simulink model "diff_drive_motion_model"  (R2018b)
settings: Solver=FixedStepDiscrete  StartTime=0.0  StopTime=10.0  FixedStep=0.01  RelTol=1e-3
values from neighbouring files (symbols this model uses):
  J = 0.02    [diff_drive_mm_workspace.m]
  K = 5    [diff_drive_mm_workspace.m]
  Kb = 0.1    [diff_drive_mm_workspace.m]
  Kf = 0.2    [diff_drive_mm_workspace.m]
  Km = 0.1    [diff_drive_mm_workspace.m]
  L = 0.5    [diff_drive_mm_workspace.m]
  R = 2.0    (= 2)    [diff_drive_mm_workspace.m]
undefined symbols (not defined in the file or in its folder): DiscIntNeverNeededParam
libraries: simulink x3
settings Model: Creator=Adhiti  LastModifiedBy=Adhiti

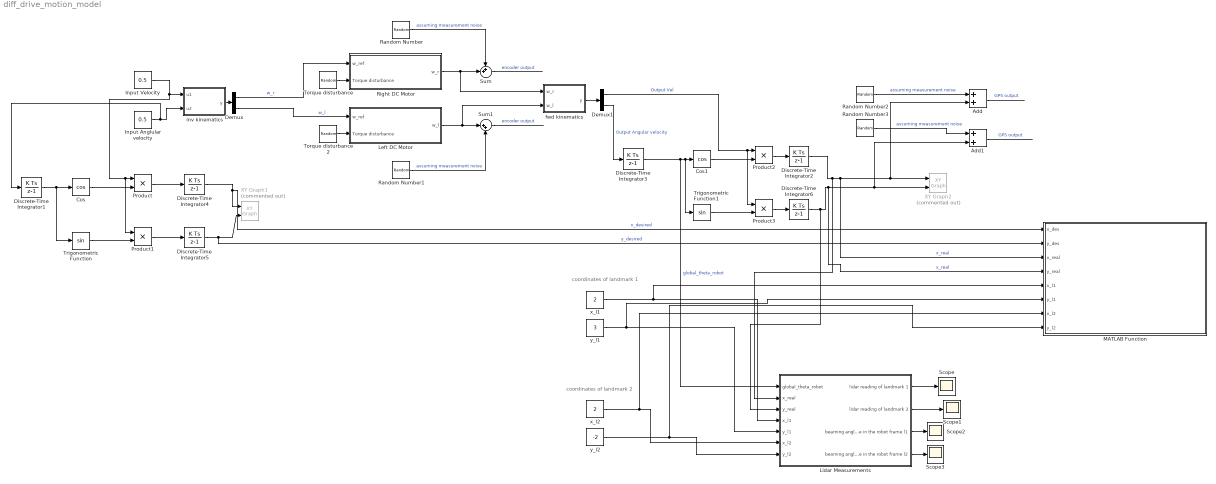
== system diff_drive_motion_model ==
  note: coordinates of landmark 2
  note: coordinates of landmark 1
  Add : Sum
  Add1 : Sum
  Cos : Trigonometry  Operator=cos
  Cos1 : Trigonometry  Operator=cos
  Demux : Demux  Outputs=2
  Demux1 : Demux  Outputs=2
  Discrete-Time Integrator{1..6} (6 alike) : DiscreteIntegrator  SampleTime=-1  ICPrevOutput=DiscIntNeverNeededParam  ICPrevScaledInput=DiscIntNeverNeededParam
  Input Anglular velocity : Constant  Value=0.5
  Input Velocity : Constant  Value=0.5
  Left DC Motor : Subsystem
  Lidar Measurements : Subsystem
  MATLAB Function : MATLAB Function  TreatAsAtomicUnit=on
  Product{,1..3} (4 alike) : Product
  Random Number{,1..3} (4 alike) : RandomNumber  Variance=0.01
  Right DC Motor : Subsystem
  Scope{,1..3} (4 alike) : Scope
  Sum : Sum  Inputs=++|
  Sum1 : Sum  Inputs=|++
  "Torque disturbance " : RandomNumber  Variance=0.0001
  Torque disturbance 2 : RandomNumber  Variance=0.0001
  Trigonometric Function : Trigonometry
  Trigonometric Function1 : Trigonometry
  XY Graph1 : simulink/Sinks/XY Graph  Commented=on  xmin=-2  xmax=2  ymin=-2  ymax=2  st=-1
  XY Graph2 : simulink/Sinks/XY Graph  Commented=on  xmin=-2  xmax=2  ymin=-2  ymax=2  st=-1
  fwd kinematics : MATLAB Function  TreatAsAtomicUnit=on
  "inv kinematics " : MATLAB Function  TreatAsAtomicUnit=on
  x_l1 : Constant  Value=2
  x_l2 : Constant  Value=2
  y_l1 : Constant  Value=3
  y_l2 : Constant  Value=-2
  wires:
  Input Anglular velocity/1 -> Discrete-Time Integrator1/1, "inv kinematics "/2(u2)
  "inv kinematics "/1(y) -> Demux/1
  Demux/2 -> Left DC Motor/1(w_ref)  "w_l"
  Demux/1 -> Right DC Motor/1(w_ref)  "w_r"
  "Torque disturbance "/1 -> Right DC Motor/2(Torque disturbance)
  Torque disturbance 2/1 -> Left DC Motor/2(Torque disturbance)
  Random Number/1 -> Sum/1  "assuming measurement noise"
  Right DC Motor/1(w_r) -> fwd kinematics/1(w_r), Sum/2
  Random Number1/1 -> Sum1/2  "assuming measurement noise"
  Left DC Motor/1(w_l) -> fwd kinematics/2(w_l), Sum1/1
  fwd kinematics/1(y) -> Demux1/1
  Demux1/1 -> Product3/1, Product2/1  "Output Vel"
  Demux1/2 -> Discrete-Time Integrator3/1  "Output Angular velocity"
  Discrete-Time Integrator1/1 -> Trigonometric Function/1, Cos/1
  Cos/1 -> Product/2
  Input Velocity/1 -> Product1/1, Product/1, "inv kinematics "/1(u1)
  Trigonometric Function/1 -> Product1/2
  Product/1 -> Discrete-Time Integrator4/1
  Product1/1 -> Discrete-Time Integrator5/1
  Product3/1 -> Discrete-Time Integrator6/1
  Trigonometric Function1/1 -> Product3/2
  Cos1/1 -> Product2/2
  Product2/1 -> Discrete-Time Integrator2/1
  Sum/1 -> ?  "encoder output"
  Sum1/1 -> ?  "encoder output"
  Discrete-Time Integrator4/1 -> MATLAB Function/1(x_des), XY Graph1/1  "x_desired"
  Discrete-Time Integrator5/1 -> MATLAB Function/2(y_des), XY Graph1/2  "y_desired"
  Discrete-Time Integrator2/1 -> Lidar Measurements/2(x_real), MATLAB Function/3(x_real), Add/2, XY Graph2/1  "x_real"
  Discrete-Time Integrator3/1 -> Lidar Measurements/1(global_theta_robot), Trigonometric Function1/1, Cos1/1  "global_theta_robot"
  x_l1/1 -> MATLAB Function/5(x_l1), Lidar Measurements/4(x_l1)
  y_l1/1 -> MATLAB Function/6(y_l1), Lidar Measurements/5(y_l1)
  x_l2/1 -> MATLAB Function/7(x_l2), Lidar Measurements/6(x_l2)
  y_l2/1 -> Lidar Measurements/7(y_l2), MATLAB Function/8(y_l2)
  Lidar Measurements/1(lidar reading of landmark 1) -> Scope/1
  Lidar Measurements/2(lidar reading of landmark 2) -> Scope1/1
  Lidar Measurements/3(bearning angle in the robot frame l1) -> Scope2/1
  Lidar Measurements/4(bearning angle in the robot frame l2) -> Scope3/1
  Random Number2/1 -> Add/1  "assuming measurement noise"
  Discrete-Time Integrator6/1 -> Lidar Measurements/3(y_real), Add1/2, XY Graph2/2, MATLAB Function/4(y_real)  "x_real"
  Random Number3/1 -> Add1/1  "assuming measurement noise"
  Add/1 -> ?  "GPS output"
  Add1/1 -> ?  "GPS output"

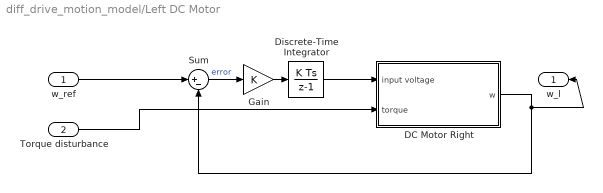
== system diff_drive_motion_model/Left DC Motor ==
  w_ref : Inport
  Torque disturbance : Inport  Port=2
  DC Motor Right : Subsystem
  Discrete-Time Integrator : DiscreteIntegrator  SampleTime=-1  ICPrevOutput=DiscIntNeverNeededParam  ICPrevScaledInput=DiscIntNeverNeededParam
  Gain : Gain  Gain=K
  Sum : Sum  Inputs=|+-
  w_l : Outport
  wires:
  Torque disturbance/1 -> DC Motor Right/2(torque)
  Gain/1 -> Discrete-Time Integrator/1
  w_ref/1 -> Sum/1
  Discrete-Time Integrator/1 -> DC Motor Right/1(input voltage)
  DC Motor Right/1(w) -> Sum/2, w_l/1
  Sum/1 -> Gain/1  "error"

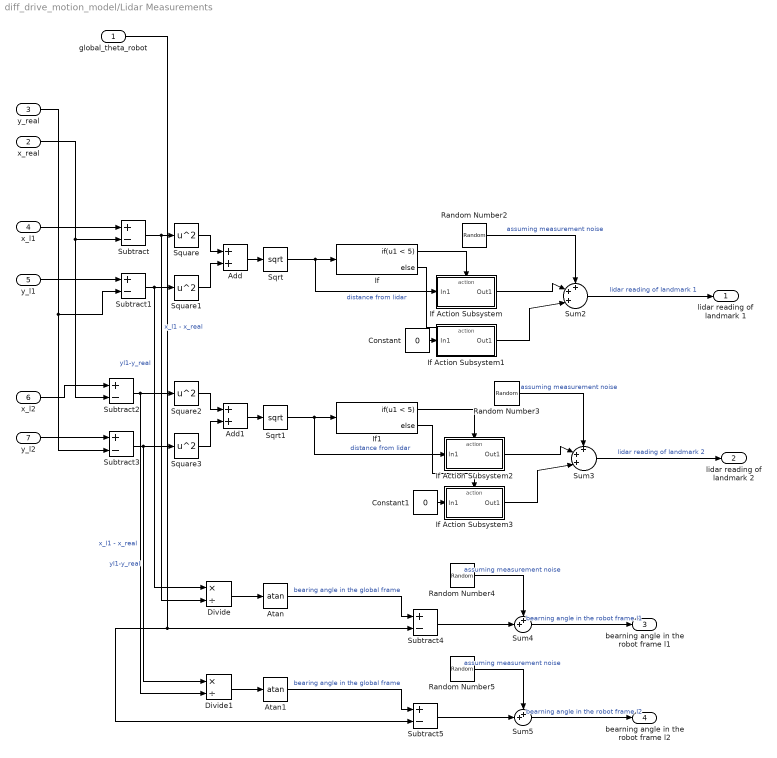
== system diff_drive_motion_model/Lidar Measurements ==
  global_theta_robot : Inport
  x_real : Inport  Port=2
  y_real : Inport  Port=3
  x_l1 : Inport  Port=4
  y_l1 : Inport  Port=5
  x_l2 : Inport  Port=6
  y_l2 : Inport  Port=7
  Add : Sum
  Add1 : Sum
  Atan : Trigonometry  Operator=atan
  Atan1 : Trigonometry  Operator=atan
  Constant : Constant  Value=0
  Constant1 : Constant  Value=0
  Divide : Product  Inputs=*/
  Divide1 : Product  Inputs=*/
  If : If  IfExpression=u1 < 5
  If Action Subsystem : Subsystem  TreatAsAtomicUnit=on
  If Action Subsystem1 : Subsystem  TreatAsAtomicUnit=on
  If Action Subsystem2 : Subsystem  TreatAsAtomicUnit=on
  If Action Subsystem3 : Subsystem  TreatAsAtomicUnit=on
  If1 : If  IfExpression=u1 < 5
  Random Number{2..5} (4 alike) : RandomNumber  Variance=0.01
  Sqrt : Sqrt  SaturateOnIntegerOverflow=on
  Sqrt1 : Sqrt  SaturateOnIntegerOverflow=on
  Square{,1..3} (4 alike) : Math  Operator=square  SaturateOnIntegerOverflow=on
  Subtract{,1..5} (6 alike) : Sum  Inputs=+-
  Sum2 : Sum  Inputs=+++|
  Sum3 : Sum  Inputs=+++|
  Sum4 : Sum  Inputs=++|
  Sum5 : Sum  Inputs=++|
  lidar reading of landmark 1 : Outport
  lidar reading of landmark 2 : Outport  Port=2
  bearning angle in the robot frame l1 : Outport  Port=3
  bearning angle in the robot frame l2 : Outport  Port=4
  wires:
  Add/1 -> Sqrt/1
  Subtract/1 -> Divide/2, Square/1  "x_l1 - x_real"
  Divide/1 -> Atan/1
  Atan/1 -> Subtract4/1  "bearing angle in the global frame"
  Divide1/1 -> Atan1/1
  If Action Subsystem3/1(Out1) -> Sum3/3
  Add1/1 -> Sqrt1/1
  Square/1 -> Add/1
  Subtract5/1 -> Sum5/2
  Random Number4/1 -> Sum4/1  "assuming measurement noise"
  Subtract1/1 -> Divide/1, Square1/1  "yl1-y_real"
  If Action Subsystem1/1(Out1) -> Sum2/3
  y_l2/1 -> Subtract3/1
  Square1/1 -> Add/2
  If/1 -> If Action Subsystem/Action
  Square3/1 -> Add1/2
  Square2/1 -> Add1/1
  Sum5/1 -> bearning angle in the robot frame l2/1  "bearning angle in the robot frame l2"
  If1/2 -> If Action Subsystem3/Action
  Sum2/1 -> lidar reading of landmark 1/1  "lidar reading of landmark 1"
  Constant1/1 -> If Action Subsystem3/1(In1)
  Subtract3/1 -> Divide1/1, Square3/1  "yl1-y_real"
  x_real/1 -> Subtract2/2, Subtract/2
  Subtract2/1 -> Divide1/2, Square2/1  "x_l1 - x_real"
  If1/1 -> If Action Subsystem2/Action
  Sum3/1 -> lidar reading of landmark 2/1  "lidar reading of landmark 2"
  y_real/1 -> Subtract1/2, Subtract3/2
  If/2 -> If Action Subsystem1/Action
  x_l1/1 -> Subtract/1
  Constant/1 -> If Action Subsystem1/1(In1)
  If Action Subsystem/1(Out1) -> Sum2/2
  y_l1/1 -> Subtract1/1
  Subtract4/1 -> Sum4/2
  global_theta_robot/1 -> Subtract5/2, Subtract4/2
  Random Number2/1 -> Sum2/1  "assuming measurement noise"
  Random Number3/1 -> Sum3/1  "assuming measurement noise"
  If Action Subsystem2/1(Out1) -> Sum3/2
  Sum4/1 -> bearning angle in the robot frame l1/1  "bearning angle in the robot frame l1"
  Random Number5/1 -> Sum5/1  "assuming measurement noise"
  Atan1/1 -> Subtract5/1  "bearing angle in the global frame"
  x_l2/1 -> Subtract2/1
  Sqrt/1 -> If Action Subsystem/1(In1), If/1  "distance from lidar"
  Sqrt1/1 -> If Action Subsystem2/1(In1), If1/1  "distance from lidar"

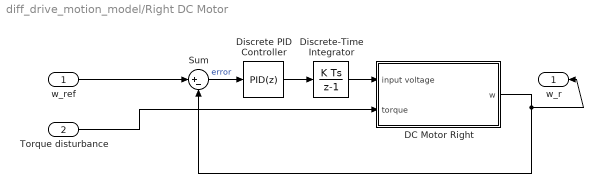
== system diff_drive_motion_model/Right DC Motor ==
  w_ref : Inport
  Torque disturbance : Inport  Port=2
  DC Motor Right : Subsystem
  Discrete PID Controller : simulink/Continuous/PID Controller  Controller=PID  Form=Parallel  TimeDomain=Discrete-time  SampleTime=-1  IntegratorMethod=Forward Euler  FilterMethod=Forward Euler  ControllerParametersSource=internal  P=1  I=1  D=0  UseFilter=on  N=100  TunerSelectOption=Transfer Function Based (PID Tuner App)  InitialConditionSource=internal  InitialConditionForIntegrator=0  InitialConditionForFilter=0  DifferentiatorICPrevScaledInput=0  ExternalReset=none  TrackingMode=off  Kt=1  LimitOutput=off  UpperSaturationLimit=inf  LowerSaturationLimit=-inf  LinearizeAsGain=off  AntiWindupMode=none  Kb=1  POutMin=[]  POutMax=[]  IOutMin=[]  IOutMax=[]  DOutMin=[]  DOutMax=[]  NOutMin=[]  NOutMax=[]  SumOutMin=[]  SumOutMax=[]  SaturationOutMin=[]  SaturationOutMax=[]  PParamMin=[]  PParamMax=[]  IParamMin=[]  IParamMax=[]  DParamMin=[]  DParamMax=[]  NParamMin=[]  NParamMax=[]  KbParamMin=[]  KbParamMax=[]  KtParamMin=[]  KtParamMax=[]  KbOutMin=[]  KbOutMax=[]  KtOutMin=[]  KtOutMax=[]  IntegratorOutMin=[]  IntegratorOutMax=[]  FilterOutMin=[]  FilterOutMax=[]  SumI1OutMin=[]  SumI1OutMax=[]  SumI2OutMin=[]  SumI2OutMax=[]  SumI3OutMin=[]  SumI3OutMax=[]  SumI4OutMin=[]  SumI4OutMax=[]  SumDOutMin=[]  SumDOutMax=[]  DifferentiatorOutMin=[]  DifferentiatorOutMax=[]  FilterDiffOutCoefMin=[]  FilterDiffOutCoefMax=[]  ReciprocalOutMin=[]  ReciprocalOutMax=[]  SumDenOutMin=[]  SumDenOutMax=[]  SumNumOutMin=[]  SumNumOutMax=[]  DivideOutMin=[]  DivideOutMax=[]  IntegratorContinuousStateAttributes=''  IntegratorStateMustResolveToSignalObject=off  IntegratorRTWStateStorageClass=Auto  FilterContinuousStateAttributes=''  FilterStateMustResolveToSignalObject=off  FilterRTWStateStorageClass=Auto  ParallelPVariant=InternalParameters  IdealPVariant=Disabled  IVariant=InternalParameters  DVariant=InternalParameters  IntegratorVariant=Discrete  SatVariant=Disabled  AWVariant=Passthrough  PCopyVariant=Disabled  TRVariant=Disabled  FdbkBlocksVariant=Forward  IdealPFdbkVariant=Disabled  SatFdbkVariant=Disabled  DerivativeFilterVariant=ForwardEulerFilter  NVariant=InternalParameters  NCopyVariant=Disabled  FilterICVariant=InternalICsFilter  IntegratorICVariant=InternalICs  ExternalResetVariant=Disabled  TRSumVariant=Passthrough  SumFdbkVariant=Disabled  SumVariant=Sum_PID
  Discrete-Time Integrator : DiscreteIntegrator  SampleTime=-1  ICPrevOutput=DiscIntNeverNeededParam  ICPrevScaledInput=DiscIntNeverNeededParam
  Sum : Sum  Inputs=|+-
  w_r : Outport
  wires:
  Torque disturbance/1 -> DC Motor Right/2(torque)
  Discrete PID Controller/1 -> Discrete-Time Integrator/1
  w_ref/1 -> Sum/1
  Discrete-Time Integrator/1 -> DC Motor Right/1(input voltage)
  DC Motor Right/1(w) -> Sum/2, w_r/1
  Sum/1 -> Discrete PID Controller/1  "error"

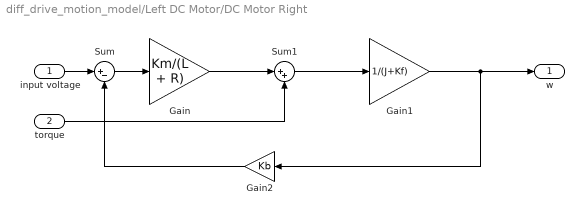
== system diff_drive_motion_model/Left DC Motor/DC Motor Right ==
  input voltage : Inport
  torque : Inport  Port=2
  Gain : Gain  Gain=Km/(L + R)
  Gain1 : Gain  Gain=1/(J+Kf)
  Gain2 : Gain  Gain=Kb
  Sum : Sum  Inputs=|+-
  Sum1 : Sum  Inputs=|++
  w : Outport
  wires:
  input voltage/1 -> Sum/1
  Sum/1 -> Gain/1
  Gain1/1 -> Gain2/1, w/1
  Sum1/1 -> Gain1/1
  Gain/1 -> Sum1/1
  Gain2/1 -> Sum/2
  torque/1 -> Sum1/2

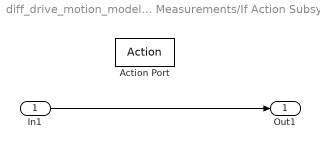
== system diff_drive_motion_model/Lidar Measurements/If Action Subsystem ==
  In1 : Inport
  Action Port : ActionPort  ActionType=then
  Out1 : Outport
  wires:
  In1/1 -> Out1/1

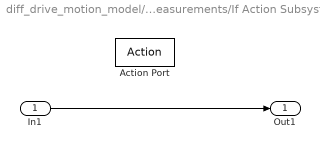
== system diff_drive_motion_model/Lidar Measurements/If Action Subsystem1 ==
  In1 : Inport
  Action Port : ActionPort  ActionType=else
  Out1 : Outport
  wires:
  In1/1 -> Out1/1

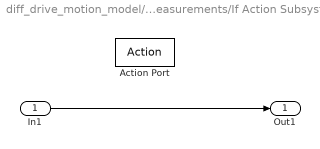
== system diff_drive_motion_model/Lidar Measurements/If Action Subsystem2 ==
  In1 : Inport
  Action Port : ActionPort  ActionType=then
  Out1 : Outport
  wires:
  In1/1 -> Out1/1

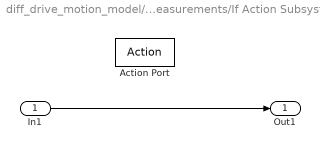
== system diff_drive_motion_model/Lidar Measurements/If Action Subsystem3 ==
  In1 : Inport
  Action Port : ActionPort  ActionType=else
  Out1 : Outport
  wires:
  In1/1 -> Out1/1

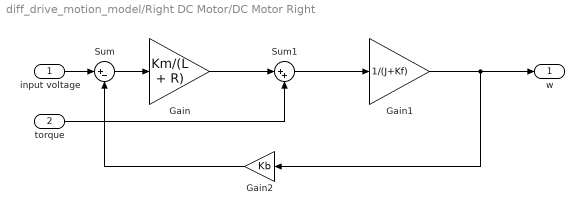
== system diff_drive_motion_model/Right DC Motor/DC Motor Right ==
  input voltage : Inport
  torque : Inport  Port=2
  Gain : Gain  Gain=Km/(L + R)
  Gain1 : Gain  Gain=1/(J+Kf)
  Gain2 : Gain  Gain=Kb
  Sum : Sum  Inputs=|+-
  Sum1 : Sum  Inputs=|++
  w : Outport
  wires:
  input voltage/1 -> Sum/1
  Sum/1 -> Gain/1
  Gain1/1 -> Gain2/1, w/1
  Sum1/1 -> Gain1/1
  Gain/1 -> Sum1/1
  Gain2/1 -> Sum/2
  torque/1 -> Sum1/2

== matlab function diff_drive_motion_model/fwd kinematics ==
  data: w_r input; y output; w_l input
function y = fcn(w_r,w_l)

    r = 1;
    length = 3;

    A = [r/2 r/2; r/length -r/length];
    
    
y = A*[w_r,w_l]';

== matlab function diff_drive_motion_model/inv kinematics  ==
  data: u1 input; y output; u2 input
function y = fcn(u1,u2)
    
    r = 1;
    length = 3;

    A = [r/2 r/2; r/length -r/length];
    
    
y = A\[u1,u2]';

== matlab function diff_drive_motion_model/MATLAB Function ==
  data: x_des input; y_des input; x_real input; y_real input; x_l1 input; y_l1 input; x_l2 input; y_l2 input
function fcn(x_des,y_des,x_real,y_real,x_l1,y_l1,x_l2,y_l2)

    plot(x_des,y_des,'.b');
    hold on;
    xlim([-5 5]);
    ylim([-5 5]);
    plot(x_real,y_real,'.r');
    plot(x_l1,y_l1,'ok',x_l2,y_l2,'ok');
